simulink model "code_gen_HeadingHold"  (Simulink 7.5)
settings: Solver=FixedStepDiscrete  SolverMode=SingleTasking  StartTime=0.0  StopTime=10.0  FixedStep=0.01  RelTol=1e-3
InitFcn:
  | boat_constants
values from neighbouring files (symbols this model uses):
  figure8_waypoints = int32([ ... (first row only)    [boat_constants.m]
  OC2max = 49999    [boat_constants.m]    (also in simulation_constants.m)
  sampling_waypoints = int32([ ... (first row only)    [boat_constants.m]
  T_step = 0.01    [boat_constants.m]    (also in common.m)
  test_waypoints = int32([ ... (first row only)    [boat_constants.m]
undefined symbols (not defined in the file or in its folder): clearGpsData, clearSensorData, cpInitCommunications, DataEEInitAndClear, DataEEWrite, DiscIntNeverNeededParam, ecan1_buffered_transmit_matlab, ecan1_error_status_matlab, ecan1_init, ecan1_receive_matlab, getGpsData, getSensorData, Init_onlyOnce, Init_Reset, initCalibrationRange, initGps, processNewCommData, processNewGpsData, setHilMode, u1, u2, uart1EnqueueStateData, uart2EnqueueActuatorData, y1
libraries: simulink x85, dsPICdrivers x44, uSimLib x6, simulink_need_slupdate x4, aerolibconvert2 x2
(part 1 of 6)
CloseFcn:
  | rtwprivate ssgencode ModelCloseRequest code_gen
settings Model: Creator=bwmairs  LastModifiedBy=Bryant  BufferReuse=off
settings OptimizationCC: InlineParams=on  InlineInvariantSignals=on  OptimizeBlockIOStorage=off  BufferReuse=off  ExpressionFolding=off  LocalBlockOutputs=off  ZeroExternalMemoryAtStartup=off  ZeroInternalMemoryAtStartup=off  NoFixptDivByZeroProtection=on  EfficientFloat2IntCast=on  OptimizeModelRefInitCode=on
settings DebuggingCC: ReadBeforeWriteMsg=DisableAll  WriteAfterWriteMsg=DisableAll  WriteAfterReadMsg=DisableAll  ParameterOverflowMsg=warning  UniqueDataStoreMsg=error
settings HardwareCC: ProdBitPerInt=16  ProdIntDivRoundTo=Zero  ProdEndianess=LittleEndian  ProdWordSize=16  ProdHWDeviceType=16-bit Generic
settings RTWCC: SystemTargetFile=dspic.tlc  MakeCommand=make_CreateMPLAB  TemplateMakefile=dspic_pic30_gcc.tmf  PostCodeGenCommand=dsPIC_Compile()  Description=Embedded Target for Microchip dsPIC (real-time)  ProcessScript=dspic_make_rtw_hook  RTWCompilerOptimization=On
settings RTWCC: CustomSource=|
  | ../../../ECAN_dspic/circBuffer.c
  | ../../../ECAN_dspic/ecanFunctions.c
  | clib/gps.c
  | clib/commProtocol.c
  | clib/uart1.c
  | clib/uart2.c
  | clib/DEE.c
  | clib/DEES.s
  | clib/misc.c
settings CodeAppCC: IgnoreCustomStorageClasses=off  IgnoreTestpoints=on
settings STFCustomTargetCC: TargetFunctionLibrary=C89/C90 (ANSI)  IncludeMdlTerminateFcn=off  CombineOutputUpdateFcns=on  SuppressErrorStatus=on  ERTCustomFileBanners=on  SupportAbsoluteTime=off  SupportNonFinite=off  SupportComplex=off  SupportContinuousTime=off  SupportNonInlinedSFcns=off  SystemTargetFile=dspic.tlc
settings ERTTargetCC: TargetFunctionLibrary=C89/C90 (ANSI)  MultiwordLength=2048  ParMdlRefBuildCompliant=off  CompOptLevelCompliant=off  IncludeMdlTerminateFcn=off  SuppressErrorStatus=on  ERTFirstTimeCompliant=off  SupportAbsoluteTime=off  SupportNonFinite=off  SupportComplex=off  ModelStepFunctionPrototypeControlCompliant=off  CPPClassGenCompliant=off  ExtModeMexFile=ext_serial_win32_comm  InlinedParameterPlacement=NonHierarchical  ERTSrcFileBannerTemplate=dsPIC_code_template.cgt  ERTHdrFileBannerTemplate=dsPIC_code_template.cgt  ERTDataSrcFileTemplate=dsPIC_code_template.cgt  ERTDataHdrFileTemplate=dsPIC_code_template.cgt  ERTCustomFileTemplate=dsPIC_main.tlc
settings CustomProperty: DataType=string  Value=C:\PROGRA~1\MATLAB\R2010a\bin\win64\gmake

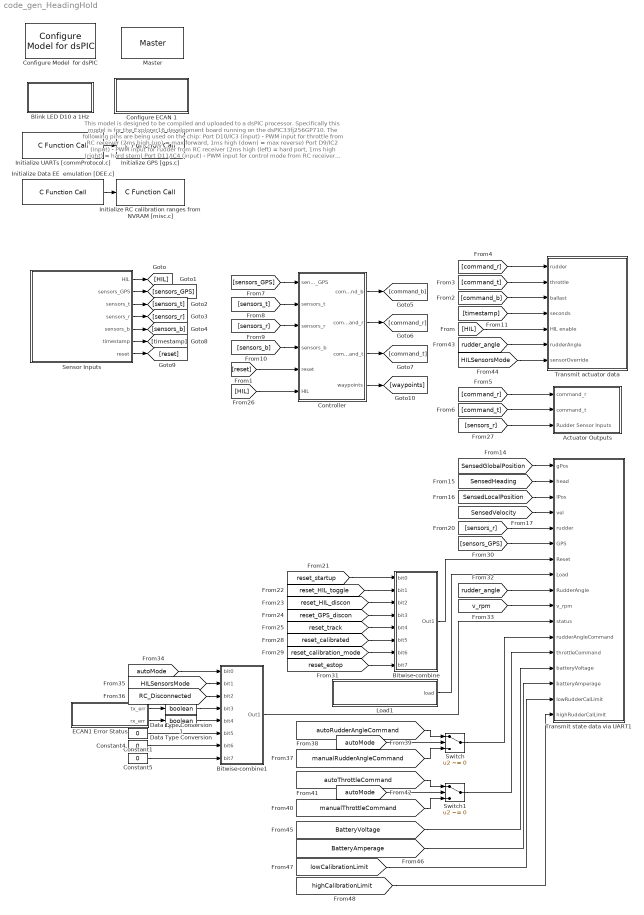
== system code_gen_HeadingHold ==
  note: This model is designed to be compiled and uploaded to a dsPIC processor.
      | Specifically this model is for the Explorer16 development board running on
      | the dsPIC33fj256GP710. The following pins are being used on the chip:
      | Port D10/IC3 (input) - PWM input for throttle from RC receiver (2ms high (up) = max forward, 1ms high (down) = max reverse)
      | Port D9/IC2 (input) - PWM input for rudder from RC receiver (2ms high (left) = hard port, 1ms high (right) = hard stern)
      | Port D11/IC4 (input) - PWM input for control mode from RC receiver (2ms high (down) = manual control, 1ms high (up) = auto. control)
      | Port D15/IC8 (input) - PWM input for track control from RC receiver (2ms high (left) = resetTrack, 1ms high (right) = nextTrack)
      | Port C2 (input) - Port hall effect sensor
      | Port G3 (input) - Starboard hall effect sensor
      | Port B4/AN4 (input) - ADC input for the TC1047 temperature sensor
      | Port B0/AN0 (input) - Potentiometer measuring position for the rudder
      | Port OC2/RD1 (output) - Step output for the rudder driver board
      | Port G9 (output) - Enable output for the rudder driver board, wired low
      | Port D5 (output) - Direction output for the rudder driver board (low = rudder turns to port)
      | Ports F0/1 (in/out) - Pins required for the ECAN1 peripheral. This is used for controlling the propeller motor.
      | Ports F4/5 (in/out) - Pins required for the UART2 peripheral. This is used for HIL data or GPS input.
      | Port A7 (out) - 1Hz pulses to blink a status LED
      | Port A0 (out) - High when in reset (drives an LED on the explorer16)
      | Port A1 (out) - High when in HIL mode (drives an LED on the explorer16)
      | Port A2 (out) - High when autonomous mode is enabled. (drives an LED on the explorer16)
      | Port F2/3 (in/out) - UART1 transmission line.
      | Port B9/11 (in/in) - ADC inputs for voltage (B9) and current (B11) sensor
      |
      | A failsafe has been implemented to detect the loss of an RC connection. It reduces propeller speed to zero and
      | disables rudder control.
      |
      | Switching between the autonomous controller and manual control involves using the landing gear channel. When
      | it's enabled, it's under autonomous control. This can only be changed when the RC transmitter is on and connected and
      | is never changed otherwise.
  Actuator Outputs : Subsystem
  Bitwise-combine : Subsystem
  Bitwise-combine1 : Subsystem
  Blink LED D10 a 1Hz : Subsystem
      mask Display: disp('blink');
  Configure ECAN 1 : Subsystem  mask(Initialize ECAN 1){frame_setting=off, mode=Normal, dma_rx_chan=2, dma_tx_chan=0, baud=250000, ps1=8, pd=5, ps2=6, sjw=4, tq=20, triple_sample=on, dma_buf_size=8 buffers, rx_bufs=[1], tx_bufs=[0], buf_0_tx_pri=Highest, buf_0_rte=No, buf_1_tx_pri=Highest, buf_1_rte=No, buf_2_tx_pri=Lowest, buf_2_rte=No, buf_3_tx_pri=Lowest, buf_3_rte=No, buf_4_tx_pri=Lowest, buf_4_rte=No, buf_5_tx_pri=Lowest, buf_5_rte=No, buf_6_tx_pri=Lowest, buf_6_rte=No, buf_7_tx_pri=Lowest, buf_7_rte=No, mask_0=0, mask_0_mide=Match std or ext, mask_1=0, mask_1_mide=Match std or ext, mask_2=0, mask_2_mide=Match std or ext, filters=[0], filter_0=0, filter_0_mask=0, filter_0_exide=Match only standard, filter_0_buf=1, filter_1=hex2dec('401'), filter_1_mask=0, filter_1_exide=Match only standard, filter_1_buf=2, filter_2=hex2dec('402'), filter_2_mask=0, filter_2_exide=Match only standard, filter_2_buf=3, filter_3=0, filter_3_mask=0, filter_3_exide=Match only standard, filter_3_buf=0, filter_4=0, filter_4_mask=0, filter_4_exide=Match only standard, filter_4_buf=0, filter_5=0, filter_5_mask=0, filter_5_exide=Match only standard, filter_5_buf=0, filter_6=0, filter_6_mask=0, filter_6_exide=Match only standard, filter_6_buf=0, filter_7=0, filter_7_mask=0, filter_7_exide=Match only standard, filter_7_buf=0, filter_8=0, filter_8_mask=0, filter_8_exide=Match only standard, filter_8_buf=0, filter_9=0, filter_9_mask=<empty>, filter_9_exide=Match only standard, filter_9_buf=0, filter_10=0, filter_10_mask=0, filter_10_exide=Match only standard, filter_10_buf=0, filter_11=0, filter_11_mask=0, filter_11_exide=Match only standard, filter_11_buf=0, filter_12=0, filter_12_mask=0, filter_12_exide=Match only standard, filter_12_buf=0, filter_13=0, filter_13_mask=0, filter_13_exide=Match only standard, filter_13_buf=0, filter_14=0, filter_14_mask=0, filter_14_exide=Match only standard, filter_14_buf=0, filter_15=0, filter_15_mask=0, filter_15_exide=Match only standard, filter_15_buf=0}
      mask prompts: frame_setting "Extended Frames (Standard if unchecked)"; dma_rx_chan "DMA Reception Channel"; dma_tx_chan "DMA Transmission Channel"; baud "Baud Rate (bps)"; ps1 "Phase Segment 1"; pd "Propagation Delay"; ps2 "Phase Segment 2"; sjw "Sync Jump Width"; tq "Time Quanta"; triple_sample "Triple-sample"; dma_buf_size "DMA Buffer Size"; rx_bufs "Reception Buffers"; tx_bufs "Transmission Buffers"; buf_0_tx_pri "Buffer 0 Transmission Priority"; buf_0_rte "Buffer 0 Remote Transmit Enable"; buf_1_tx_pri "Buffer 1 Transmission Priority"; buf_1_rte "Buffer 1 Remote Transmit Enable"; buf_2_tx_pri "Buffer 2 Transmission Priority"; buf_2_rte "Buffer 2 Remote Transmit Enable"; buf_3_tx_pri "Buffer 3 Transmission Priority"; buf_3_rte "Buffer 3 Remote Transmit Enable"; buf_4_tx_pri "Buffer 4 Transmission Priority"; buf_4_rte "Buffer 4 Remote Transmit Enable"; buf_5_tx_pri "Buffer 5 Transmission Priority"; buf_5_rte "Buffer 5 Remote Transmit Enable"; buf_6_tx_pri "Buffer 6 Transmission Priority"; buf_6_rte "Buffer 6 Remote Transmit Enable"; buf_7_tx_pri "Buffer 7 Transmission Priority"; buf_7_rte "Buffer 7 Remote Transmit Enable"; mask_0 "Mask 0"; mask_0_mide "Mask 0 Receive Mode"; mask_1 "Mask 1"; mask_1_mide "Mask 1 Receive Mode"; mask_2 "Mask 2"; mask_2_mide "Mask 2 Receive Mode"; filter_0 "Filter 0"; filter_0_mask "Filter 0 Mask"; filter_0_exide "Filter 0 Mode"; filter_0_buf "Filter 0 Buffer"; filter_1 "Filter 1"; filter_1_mask "Filter 1 Mask"; filter_1_exide "Filter 1 Mode"; filter_1_buf "Filter 1 Buffer"; filter_2 "Filter 2"; filter_2_mask "Filter 2 Mask"; filter_2_exide "Filter 2 Mode"; filter_2_buf "Filter 2 Buffer"; filter_3 "Filter 3"; filter_3_mask "Filter 3 Mask"; filter_3_exide "Filter 3 Mode"; filter_3_buf "Filter 3 Buffer"; filter_4 "Filter 4"; filter_4_mask "Filter 4 Mask"; filter_4_exide "Filter 4 Mode"; filter_4_buf "Filter 4 Buffer"; filter_5 "Filter 5"; filter_5_mask "Filter 5 Mask"; filter_5_exide "Filter 5 Mode"; filter_5_buf "Filter 5 Buffer"; filter_6 "Filter 6"; filter_6_mask "Filter 6 Mask"; filter_6_exide "Filter 6 Mode"; filter_6_buf "Filter 6 Buffer"; filter_7 "Filter 7"; filter_7_mask "Filter 7 Mask"; filter_7_exide "Filter 7 Mode"; filter_7_buf "Filter 7 Buffer"; filter_8 "Filter 8"; filter_8_mask "Filter 8 Mask"; filter_8_exide "Filter 8 Mode"; filter_8_buf "Filter 8 Buffer"; filter_9 "Filter 9"; filter_9_mask "Filter 9 Mask"; filter_9_exide "Filter 9 Mode"; filter_9_buf "Filter 9 Buffer"; filter_10 "Filter 10"; filter_10_mask "Filter 10 Mask"; filter_10_exide "Filter 10 Mode"; filter_10_buf "Filter 10 Buffer"; filter_11 "Filter 11"; filter_11_mask "Filter 11 Mask"; filter_11_exide "Filter 11 Mode"; filter_11_buf "Filter 11 Buffer"; filter_12 "Filter 12"; filter_12_mask "Filter 12 Mask"; filter_12_exide "Filter 12 Mode"; filter_12_buf "Filter 12 Buffer"; filter_13 "Filter 13"; filter_13_mask "Filter 13 Mask"; filter_13_exide "Filter 13 Mode"; filter_13_buf "Filter 13 Buffer"; filter_14 "Filter 14"; filter_14_mask "Filter 14 Mask"; filter_14_exide "Filter 14 Mode"; filter_14_buf "Filter 14 Buffer"; filter_15 "Filter 15"; filter_15_mask "Filter 15 Mask"; filter_15_exide "Filter 15 Mode"; filter_15_buf "Filter 15 Buffer"
      mask help: Initializes the ECAN 1 module on the dsPIC33f. Allows for configuration of almost all ECAN options to produce a usable system.
      mask init:
      | parameters = uint16(zeros(53,1));
      | 
      | %% Generate parameter 1
      | parameters(1) = frame_setting;
      | mode_id = 0;
      | switch mode
      |     case 'Disabled'
      |         mode_id = 1;
      |     case 'Loopback'
      |         mode_id = 2;
      |     case 'Listen only'
      |         mode_id = 3;
      |     case 'Listen all'
      |         mode_id = 7;
      | end
      | parameters(1) = bitor(parameters(1), bitshift(mode_id, 2));
      | parameters(1) = bitor(parameters(1), bitshift(dma_rx_chan, 5));
      | parameters(1) = bitor(parameters(1), bitshift(dma_tx_chan, 8));
      | 
      | %% Generate parameter 2
      | parameters(2) = baud / 100;
      | 
      | %% Generate parameter 3
      | h = find_system(bdroot(gcb),'FollowLinks','on','LookUnderMasks','all','Tag','dsPIC_MASTER');
      | fcy = 0;
      | if ~isempty(h)
      |     %OverrideFcy = strcmp(get_param(h{1},'OverrideFcy'),'on');
      |     %if (OverrideFcy == 1)
      |     %    fcy = str2num(get_param(h{1},'NewFcy'));     %% overridded fcy
      |     %else
      |         fcy = str2num(get_param(h{1},'fcy'));
      |     %end 
      | end
      | parameters(3) = fcy / 1000;
      | 
      | %% Generate parameter 4
      | parameters(4) = ps1 - 1;
      | parameters(4) = bitor(parameters(4), bitshift(pd - 1, 3));
      | parameters(4) = bitor(parameters(4), bitshift(ps2 - 1, 6));
      | parameters(4) = bitor(parameters(4), bitshift(sjw - 1, 9));
      | if triple_sample == 1
      |     parameters(4) = bitset(parameters(4),12);
      | end
      | 
      | %% Generate parameter 5
      | for k = 1:length(filters)
      |     parameters(5) = bitset(parameters(5),filters(k)+1);
      | end;
      | 
      | % Map filter mask values into proper values
      | filter_masks = [filter_0_mask; filter_1_mask; filter_2_mask; filter_3_mask; filter_4_mask; filter_5_mask; filter_6_mask; filter_7_mask; filter_8_mask; filter_9_mask; filter_10_mask; filter_11_mask; filter_12_mask; filter_13_mask; filter_14_mask; filter_15_mask;];
      | filter_masks = filter_masks - 2;
      | filter_masks(filter_masks == -1) = 3;
      | 
      | %% Generate parameters 6 and 7
      | for k = 1:length(filters);
      |     filter = filters(k) + 1;
      |     if filter < 9
      |         parameters(6) = bitor(parameters(6), bitshift(filter_masks(filter),2*(filter-1)));
      |     else
      |         parameters(7) = bitor(parameters(7), bitshift(filter_masks(filter),2*(filter-9)));
      |     end
      | end
      | 
      | % Generate parameters 8 and 9
      | parameters(8) = bitshift(bitand(mask_0,hex2dec('18000000')),-27); % EID17-16
      | parameters(8) = bitor(parameters(8), bitshift(bitand(mask_0,hex2dec('7FF')), 5)); % SID
      | parameters(8) = bitor(parameters(8), bitshift(mask_0_mide - 1, 3)); % MIDE
      | parameters(9) = bitshift(bitand(mask_0,hex2dec('7FFF800')),-11); % EID15-0
      | 
      | %% Generate parameters 10 and 11
      | parameters(10) = bitshift(bitand(mask_1,hex2dec('18000000')),-27); % EID17-16
      | parameters(10) = bitor(parameters(10), bitshift(bitand(mask_1,hex2dec('7FF')), 5)); % SID
      | parameters(10) = bitor(parameters(10), bitshift(mask_1_mide - 1, 3)); % MIDE
      | parameters(11) = bitshift(bitand(mask_1,hex2dec('7FFF800')),-11); % EID15-0
      | 
      | %% Generate parameters 12 and 13
      | parameters(12) = bitshift(bitand(mask_2,hex2dec('18000000')),-27); % EID17-16
      | parameters(12) = bitor(parameters(12), bitshift(bitand(mask_2,hex2dec('7FF')), 5)); % SID
      | parameters(12) = bitor(parameters(12), bitshift(mask_2_mide - 1, 3)); % MIDE
      | parameters(13) = bitshift(bitand(mask_2,hex2dec('7FFF800')),-11); % EID15-0
      | 
      | % Generate parameters 14-17
      | buf_priorities = [buf_0_tx_pri;buf_1_tx_pri;buf_2_tx_pri;buf_3_tx_pri;buf_4_tx_pri;buf_5_tx_pri;buf_6_tx_pri;buf_7_tx_pri] - 1;
      | buf_rtes = [buf_0_rte;buf_1_rte;buf_2_rte;buf_3_rte;buf_4_rte;buf_5_rte;buf_6_rte;buf_7_rte] - 1;
      | 
      | % Create a vector of chars to modify
      | regs = uint16(zeros(8,1));
      | 
      | % Go through all enabled transmission buffers setting appropriate bits
      | for b = 1:size(tx_bufs,1)
      |     
      |     index = tx_bufs(b) + 1;
      |     
      |     % Set transmission bit
      |     regs(index) = bitset(regs(index),8);
      | 
      |     % Set priority bits
      |     regs(index) = bitor(regs(index), buf_priorities(index));
      | 
      |     % Set remote transmit enable bits
      |     if buf_rtes(index) == 1
      |         regs(index) = bitset(regs(index),3);
      |     end
      | end
      | 
      | for b = 1:size(rx_bufs,1)
      |     
      |     index = rx_bufs(b) + 1;
      | 
      |     % Set priority bits
      |     regs(index) = bitor(regs(index), buf_priorities(index));
      | 
      |     % Set remote transmit enable bits
      |     if buf_rtes(index) == 1
      |         regs(index) = bitset(regs(index),3);
      |     end
      | end
      | 
      | % Map our matrix into registers
      | parameters(14) = bitor(bitshift(regs(2),8), regs(1));
      | parameters(15) = bitor(bitshift(regs(4),8), regs(3));
      | parameters(16) = bitor(bitshift(regs(6),8), regs(5));
      | parameters(17) = bitor(bitshift(regs(8),8), regs(7));
      | 
      | % Map the filter buffer values to corresponding bit values
      | filter_buffers = [filter_0_buf; filter_1_buf; filter_2_buf; filter_3_buf; filter_4_buf; filter_5_buf; filter_6_buf; filter_7_buf; filter_8_buf; filter_9_buf; filter_10_buf; filter_11_buf; filter_12_buf; filter_13_buf; filter_14_buf; filter_15_buf;];
      | filter_buffers = filter_buffers - 1;
      | 
      | %% Generate parameter 18
      | if bitget(parameters(5),1) == 1
      |     parameters(18) = filter_buffers(1);
      | end
      | if bitget(parameters(5),2) == 1
      |     parameters(18) = bitor(parameters(18), bitshift(filter_buffers(2), 4));
      | end
      | if bitget(parameters(5),3) == 1
      |     parameters(18) = bitor(parameters(18), bitshift(filter_buffers(3), 8));
      | end
      | if bitget(parameters(5),4) == 1
      |     parameters(18) = bitor(parameters(18), bitshift(filter_buffers(4), 12));
      | end
      | 
      | %% Generate parameter 19
      | if bitget(parameters(5),5) == 1
      |     parameters(19) = filter_buffers(5);
      | end
      | if bitget(parameters(5),6) == 1
      |     parameters(19) = bitor(parameters(19), bitshift(filter_buffers(6), 4));
      | end
      | if bitget(parameters(5),7) == 1
      |     parameters(19) = bitor(parameters(19), bitshift(filter_buffers(7), 8));
      | end
      | if bitget(parameters(5),8) == 1
      |     parameters(19) = bitor(parameters(19), bitshift(filter_buffers(8), 12));
      | end
      | 
      | %% Generate parameter 20
      | if bitget(parameters(5),9) == 1
      |     parameters(20) = filter_buffers(9);
      | end
      | if bitget(parameters(5),10) == 1
      |     parameters(20) = bitor(parameters(20), bitshift(filter_buffers(10), 4));
      | end
      | if bitget(parameters(5),11) == 1
      |     parameters(20) = bitor(parameters(20), bitshift(filter_buffers(11), 8));
      | end
      | if bitget(parameters(5),12) == 1
      |     parameters(20) = bitor(parameters(20), bitshift(filter_buffers(12), 12));
      | end
      | 
      | %% Generate parameter 21
      | if bitget(parameters(5),13) == 1
      |     parameters(21) = filter_buffers(13);
      | end
      | if bitget(parameters(5),14) == 1
      |     parameters(21) = bitor(parameters(21), bitshift(filter_buffers(14), 4));
      | end
      | if bitget(parameters(5),15) == 1
      |     parameters(21) = bitor(parameters(21), bitshift(filter_buffers(15), 8));
      | end
      | if bitget(parameters(5),16) == 1
      |     parameters(21) = bitor(parameters(21), bitshift(filter_buffers(16), 12));
      | end
      | 
      | % Generate parameters 22 and 23
      | parameters(22) = bitshift(bitand(filter_0,hex2dec('18000000')),-27); % EID17-16
      | parameters(22) = bitor(parameters(22), bitshift(bitand(filter_0,hex2dec('7FF')), 5)); % SID
      | parameters(22) = bitor(parameters(22), bitshift(filter_0_exide - 1, 3)); % EXIDE
      | parameters(23) = bitshift(bitand(uint32(filter_0),hex2dec('7FFF800')),-11); % EID15-0
      | 
      | %% Generate parameters 24 and 25
      | parameters(24) = bitshift(bitand(filter_1,hex2dec('18000000')),-27); % EID17-16
      | parameters(24) = bitor(parameters(24), bitshift(bitand(filter_1,hex2dec('7FF')), 5)); % SID
      | parameters(24) = bitor(parameters(24), bitshift(filter_1_exide - 1, 3)); % EXIDE
      | parameters(25) = bitshift(bitand(uint32(filter_1),hex2dec('7FFF800')),-11); % EID15-0
      | 
      | %% Generate parameters 26 and 27
      | parameters(26) = bitshift(bitand(filter_2,hex2dec('18000000')),-27); % EID17-16
      | parameters(26) = bitor(parameters(26), bitshift(bitand(filter_2,hex2dec('7FF')), 5)); % SID
      | parameters(26) = bitor(parameters(26), bitshift(filter_2_exide - 1, 3)); % EXIDE
      | parameters(27) = bitshift(bitand(uint32(filter_2),hex2dec('7FFF800')),-11); % EID15-0
      | 
      | %% Generate parameters 28 and 29
      | parameters(28) = bitshift(bitand(filter_3,hex2dec('18000000')),-27); % EID17-16
      | parameters(28) = bitor(parameters(28), bitshift(bitand(filter_3,hex2dec('7FF')), 5)); % SID
      | parameters(28) = bitor(parameters(28), bitshift(filter_3_exide - 1, 3)); % EXIDE
      | parameters(29) = bitshift(bitand(uint32(filter_3),hex2dec('7FFF800')),-11); % EID15-0
      | 
      | %% Generate parameters 30 and 31
      | parameters(30) = bitshift(bitand(filter_4,hex2dec('18000000')),-27); % EID17-16
      | parameters(30) = bitor(parameters(30), bitshift(bitand(filter_4,hex2dec('7FF')), 5)); % SID
      | parameters(30) = bitor(parameters(30), bitshift(filter_4_exide - 1, 3)); % EXIDE
      | parameters(31) = bitshift(bitand(uint32(filter_4),hex2dec('7FFF800')),-11); % EID15-0
      | 
      | %% Generate parameters 32 and 33
      | parameters(32) = bitshift(bitand(filter_5,hex2dec('18000000')),-27); % EID17-16
      | parameters(32) = bitor(parameters(32), bitshift(bitand(filter_5,hex2dec('7FF')), 5)); % SID
      | parameters(32) = bitor(parameters(32), bitshift(filter_5_exide - 1, 3)); % EXIDE
      | parameters(33) = bitshift(bitand(uint32(filter_5),hex2dec('7FFF800')),-11); % EID15-0
      | 
      | %% Generate parameters 34 and 35
      | parameters(34) = bitshift(bitand(filter_6,hex2dec('18000000')),-27); % EID17-16
      | parameters(34) = bitor(parameters(34), bitshift(bitand(filter_6,hex2dec('7FF')), 5)); % SID
      | parameters(34) = bitor(parameters(34), bitshift(filter_6_exide - 1, 3)); % EXIDE
      | parameters(35) = bitshift(bitand(uint32(filter_6),hex2dec('7FFF800')),-11); % EID15-0
      | 
      | %% Generate parameters 36 and 37
      | parameters(36) = bitshift(bitand(filter_7,hex2dec('18000000')),-27); % EID17-16
      | parameters(36) = bitor(parameters(36), bitshift(bitand(filter_7,hex2dec('7FF')), 5)); % SID
      | parameters(36) = bitor(parameters(36), bitshift(filter_7_exide - 1, 3)); % EXIDE
      | parameters(37) = bitshift(bitand(uint32(filter_7),hex2dec('7FFF800')),-11); % EID15-0
      | 
      | %% Generate parameters 38 and 39
      | parameters(38) = bitshift(bitand(filter_8,hex2dec('18000000')),-27); % EID17-16
      | parameters(38) = bitor(parameters(38), bitshift(bitand(filter_8,hex2dec('7FF')), 5)); % SID
      | parameters(38) = bitor(parameters(38), bitshift(filter_8_exide - 1, 3)); % EXIDE
      | parameters(39) = bitshift(bitand(uint32(filter_8),hex2dec('7FFF800')),-11); % EID15-0
      | 
      | %% Generate parameters 40 and 41
      | parameters(40) = bitshift(bitand(filter_9,hex2dec('18000000')),-27); % EID17-16
      | parameters(40) = bitor(parameters(40), bitshift(bitand(filter_9,hex2dec('7FF')), 5)); % SID
      | parameters(40) = bitor(parameters(40), bitshift(filter_9_exide - 1, 3)); % EXIDE
      | parameters(41) = bitshift(bitand(uint32(filter_9),hex2dec('7FFF800')),-11); % EID15-0
      | 
      | %% Generate parameters 42 and 43
      | parameters(42) = bitshift(bitand(filter_10,hex2dec('18000000')),-27); % EID17-16
      | parameters(42) = bitor(parameters(42), bitshift(bitand(filter_10,hex2dec('7FF')), 5)); % SID
      | parameters(42) = bitor(parameters(42), bitshift(filter_10_exide - 1, 3)); % EXIDE
      | parameters(43) = bitshift(bitand(uint32(filter_10),hex2dec('7FFF800')),-11); % EID15-0
      | 
      | %% Generate parameters 44 and 45
      | parameters(44) = bitshift(bitand(filter_11,hex2dec('18000000')),-27); % EID17-16
      | parameters(44) = bitor(parameters(44), bitshift(bitand(filter_11,hex2dec('7FF')), 5)); % SID
      | parameters(44) = bitor(parameters(44), bitshift(filter_11_exide - 1, 3)); % EXIDE
      | parameters(45) = bitshift(bitand(uint32(filter_11),hex2dec('7FFF800')),-11); % EID15-0
      | 
      | %% Generate parameters 46 and 47
      | parameters(46) = bitshift(bitand(filter_12,hex2dec('18000000')),-27); % EID17-16
      | parameters(46) = bitor(parameters(46), bitshift(bitand(filter_12,hex2dec('7FF')), 5)); % SID
      | parameters(46) = bitor(parameters(46), bitshift(filter_12_exide - 1, 3)); % EXIDE
      | parameters(47) = bitshift(bitand(uint32(filter_12),hex2dec('7FFF800')),-11); % EID15-0
      | 
      | %% Generate parameters 48 and 49
      | parameters(48) = bitshift(bitand(filter_13,hex2dec('18000000')),-27); % EID17-16
      | parameters(48) = bitor(parameters(48), bitshift(bitand(filter_13,hex2dec('7FF')), 5)); % SID
      | parameters(48) = bitor(parameters(48), bitshift(filter_13_exide - 1, 3)); % EXIDE
      | parameters(49) = bitshift(bitand(uint32(filter_13),hex2dec('7FFF800')),-11); % EID15-0
      | 
      | %% Generate parameters 50 and 51
      | parameters(50) = bitshift(bitand(filter_14,hex2dec('18000000')),-27); % EID17-16
      | parameters(50) = bitor(parameters(50), bitshift(bitand(filter_14,hex2dec('7FF')), 5)); % SID
      | parameters(50) = bitor(parameters(50), bitshift(filter_14_exide - 1, 3)); % EXIDE
      | parameters(51) = bitshift(bitand(uint32(filter_14),hex2dec('7FFF800')),-11); % EID15-0
      | 
      | %% Generate parameters 52 and 53
      | parameters(52) = bitshift(bitand(filter_15,hex2dec('18000000')),-27); % EID17-16
      | parameters(52) = bitor(parameters(52), bitshift(bitand(filter_15,hex2dec('7FF')), 5)); % SID
      | parameters(52) = bitor(parameters(52), bitshift(filter_15_exide - 1, 3)); % EXIDE
      | parameters(53) = bitshift(bitand(uint32(filter_15),hex2dec('7FFF800')),-11); % EID15-0
      mask StyleString: checkbox,popup(Disabled|Listen all|Listen only|Loopback|Normal),edit,edit,edit,edit,edit,edit,popup(1|2|3|4),edit,checkbox,popup(4 buffers|6 buffers|8 buffers|12 buffers|16 buffers|24 buffers|32 buffers),edit,edit,popup(Lowest|Low|High|Highest),popup(No|Yes),popup(Lowest|Low|High|Highest),popup(No|Yes),popup(Lowest|Low|High|Highest),popup(No|Yes),popup(Lowest|Low|High|Highest),popup(No|Yes),popup(Lowest|Low|High|Highest),popup(No|Yes),popup(Lowest|Low|High|Highest),popup(No|Yes),popup(Lowest|Low|High|Highest),popup(No|Yes),popup(Lowest|Low|High|Highest),popup(No|Yes),edit,popup(Match std or ext|Obey filter mode),edit,popup(Match std or ext|Obey filter mode),edit,popup(Match std or ext|Obey filter mode),edit,edit,popup(--|0|1|2),popup(Match only standard|Match only extended),popup(0|1|2|3|4|5|6|7|8|9|10|11|12|13|14|FIFO),edit,popup(--|0|1|2),popup(Match only standard|Match only extended),popup(0|1|2|3|4|5|6|7|8|9|10|11|12|13|14|FIFO),edit,popup(--|0|1|2),popup(Match only standard|Match only extended),popup(0|1|2|3|4|5|6|7|8|9|10|11|12|13|14|FIFO),edit,popup(--|0|1|2),popup(Match only standard|Match only extended),popup(0|1|2|3|4|5|6|7|8|9|10|11|12|13|14|FIFO),edit,popup(--|0|1|2),popup(Match only standard|Match only extended),popup(0|1|2|3|4|5|6|7|8|9|10|11|12|13|14|FIFO),edit,popup(--|0|1|2),popup(Match only standard|Match only extended),popup(0|1|2|3|4|5|6|7|8|9|10|11|12|13|14|FIFO),edit,popup(--|0|1|2),popup(Match only standard|Match only extended),popup(0|1|2|3|4|5|6|7|8|9|10|11|12|13|14|FIFO),edit,popup(--|0|1|2),popup(Match only standard|Match only extended),popup(0|1|2|3|4|5|6|7|8|9|10|11|12|13|14|FIFO),edit,popup(--|0|1|2),popup(Match only standard|Match only extended),popup(0|1|2|3|4|5|6|7|8|9|10|11|12|13|14|FIFO),edit,popup(<empty>),popup(Match only standard|Match only extended),popup(0|1|2|3|4|5|6|7|8|9|10|11|12|13|14|FIFO),edit,popup(--|0|1|2),popup(Match only standard|Match only extended),popup(0|1|2|3|4|5|6|7|8|9|10|11|12|13|14|FIFO),edit,popup(--|0|1|2),popup(Match only standard|Match only extended),popup(0|1|2|3|4|5|6|7|8|9|10|11|12|13|14|FIFO),edit,popup(--|0|1|2),popup(Match only standard|Match only extended),popup(0|1|2|3|4|5|6|7|8|9|10|11|12|13|14|FIFO),edit,popup(--|0|1|2),popup(Match only standard|Match only extended),popup(0|1|2|3|4|5|6|7|8|9|10|11|12|13|14|FIFO),edit,popup(--|0|1|2),popup(Match only standard|Match only extended),popup(0|1|2|3|4|5|6|7|8|9|10|11|12|13|14|FIFO),edit,popup(--|0|1|2),popup(Match only standard|Match only extended),popup(0|1|2|3|4|5|6|7|8|9|10|11|12|13|14|FIFO)
      mask CallbackString:
      | |||||tq = 1 + str2num(get_param(gcb, 'ps1')) + str2num(get_param(gcb, 'pd')) + str2num(get_param(gcb, 'ps2'));
      | set_param(gcb, 'tq', int2str(tq));|tq = 1 + str2num(get_param(gcb, 'ps1')) + str2num(get_param(gcb, 'pd')) + str2num(get_param(gcb, 'ps2'));
      | set_param(gcb, 'tq', int2str(tq));|tq = 1 + str2num(get_param(gcb, 'ps1')) + str2num(get_param(gcb, 'pd')) + str2num(get_param(gcb, 'ps2'));
      | set_param(gcb, 'tq', int2str(tq));||||||filters = eval(get_param(gcb,'tx_bufs'));
      | mVisibilities = get_param(gcb,'MaskVisibilities');
      | mNames = get_param(gcb,'MaskNames');
      | for i = 1:size(mNames);
      | 	n = mNames{i};
      |     if size(n,2) > 4 && strcmp(n(1:4), 'buf_') == 1
      |         filterNumber = sscanf(n, 'buf_%d');
      |         if isempty(find(filters == filterNumber, 1)) == 0
      |              mVisibilities{i} = 'on';
      |         else
      |              mVisibilities{i} = 'off';
      |         end
      |     end
      | end
      | set_param(gcb, 'MaskVisibilities', mVisibilities);|||||||||||||||||||||||filters = eval(get_param(gcb,'filters'));
      | mVisibilities = get_param(gcb,'MaskVisibilities');
      | mNames = get_param(gcb,'MaskNames');
      | for i = 1:size(mNames);
      | 	n = mNames{i};
      |     if size(n,2) > 7 && strcmp(n(1:7), 'filter_') == 1
      |         filterNumber = sscanf(n, 'filter_%d');
      |         if isempty(find(filters == filterNumber, 1)) == 0
      |              mVisibilities{i} = 'on';
      |         else
      |              mVisibilities{i} = 'off';
      |         end
      |     end
      | end
      | set_param(gcb, 'MaskVisibilities', mVisibilities);||||||||||||||||||||||||||||||||||||||||||||||||||||||||||||||||
      mask Display: text(0.5,0.5,'Configure ECAN1','horizontalAlignment','center','verticalAlignment','middle');
  Configure Model  for dsPIC : dsPICdrivers/Simulink Configuration/Configure Model  for dsPIC
  Constant1 : Constant  Value=0  OutDataTypeMode=uint8  OutDataType=fixdt(1, 16)  OutScaling=2^0  OutDataTypeStr=uint8
  Constant4 : Constant  Value=0  OutDataTypeMode=uint8  OutDataType=fixdt(1, 16)  OutScaling=2^0  OutDataTypeStr=uint8
  Constant5 : Constant  Value=0  OutDataTypeMode=uint8  OutDataType=fixdt(1, 16)  OutScaling=2^0  OutDataTypeStr=uint8
  Controller : Subsystem
  Data Type Conversion : DataTypeConversion  OutDataTypeMode=boolean  OutDataType=fixdt(1, 16)  OutScaling=2^0  OutDataTypeStr=boolean
  Data Type Conversion1 : DataTypeConversion  OutDataTypeMode=boolean  OutDataType=fixdt(1, 16)  OutScaling=2^0  OutDataTypeStr=boolean
  ECAN1 Error Status : Subsystem  mask(ECAN 1 Reception Block){ecan1_error_sample_time=.01}
      mask prompts: ecan1_error_sample_time "Sampling time"
      mask help:
      | This block will receive CAN messages over the ECAN1 peripheral on the dsPIC33f.
      | Outputs:
      | identifier - uint32 containing SID and EID
      | data - Variable-sized array (between 0 and 8) of uint8s
      | remote - boolean value specifying if this is a remote transmit request
      mask Display: disp('ECAN1 ERR');
  Initialize Data EE  emulation [DEE.c] : dsPICdrivers/OTHERS/C Function Call  Tag=dsPIC_dsPIC_CFunctionCall  FctUpdate=None  fctName='DataEEInitAndClear'  INPUT_SIZE=1  INPUT1=--  INPUT2=--  INPUT3=--  OUTPUT_SIZE=1  OUTPUT1=--  SampleTime=Inf  InputType=[]  OutputType=[]  FctDeclaration=extern void DataEEInitAndClear();  FctCall=DataEEInitAndClear();  OrderingInOutPopup=Output  FctStart=Start Function (Call once and only once)  FctStart_Name=DataEEInitAndClear  FctStart_Declaration=inline extern void DataEEInitAndClear();  FctStart_Call=DataEEInitAndClear();  FctInit=None  FctInit_Name=Init_Reset  FctInit_Declaration=inline extern void Init_Reset();  FctInit_Call=Init_Reset();  PinDigitalInput=[]  PinDigitalOutput=[]  AnalogueInput=[]
  Initialize GPS [gps.c] : dsPICdrivers/OTHERS/C Function Call  Tag=dsPIC_dsPIC_CFunctionCall  FctUpdate=None  fctName='initGps'  INPUT_SIZE=1  INPUT1=--  INPUT2=--  INPUT3=--  OUTPUT_SIZE=1  OUTPUT1=--  SampleTime=Inf  InputType=[]  OutputType=[]  FctDeclaration=extern void initGps();  FctCall=initGps();  OrderingInOutPopup=Input  FctStart=Start Function (Call once and only once)  FctStart_Name=initGps  FctStart_Declaration=inline extern void initGps();  FctStart_Call=initGps();  FctInit=None  FctInit_Name=Init_Reset  FctInit_Declaration=inline extern void Init_Reset();  FctInit_Call=Init_Reset();  PinDigitalInput=[]  PinDigitalOutput=[]  AnalogueInput=[]
  Initialize RC calibration ranges from NVRAM [misc.c] : dsPICdrivers/OTHERS/C Function Call  Tag=dsPIC_dsPIC_CFunctionCall  FctUpdate=None  fctName='initCalibrationRange'  INPUT_SIZE=1  INPUT1=--  INPUT2=--  INPUT3=--  OUTPUT_SIZE=1  OUTPUT1=--  SampleTime=Inf  InputType=[]  OutputType=[]  FctDeclaration=extern void initCalibrationRange();  FctCall=initCalibrationRange();  OrderingInOutPopup=Input  FctStart=Start Function (Call once and only once)  FctStart_Name=initCalibrationRange  FctStart_Declaration=inline extern void initCalibrationRange();  FctStart_Call=initCalibrationRange();  FctInit=None  FctInit_Name=Init_Reset  FctInit_Declaration=inline extern void Init_Reset();  FctInit_Call=Init_Reset();  PinDigitalInput=[]  PinDigitalOutput=[]  AnalogueInput=[]
  Initialize UARTs [commProtocol.c] : dsPICdrivers/OTHERS/C Function Call  Tag=dsPIC_dsPIC_CFunctionCall  FctUpdate=None  fctName=cpInitCommunications  INPUT_SIZE=1  INPUT1=--  INPUT2=--  INPUT3=--  OUTPUT_SIZE=1  OUTPUT1=--  SampleTime=Inf  InputType=[]  OutputType=[]  FctDeclaration=extern void cpInitCommunications();  FctCall=cpInitCommunications();  OrderingInOutPopup=Output  FctStart=Start Function (Call once and only once)  FctStart_Name=cpInitCommunications  FctStart_Declaration=inline extern void cpInitCommunications();  FctStart_Call=cpInitCommunications();  FctInit=None  FctInit_Name=Init_Reset  FctInit_Declaration=inline extern void Init_Reset();  FctInit_Call=Init_Reset();  PinDigitalInput=[]  PinDigitalOutput=[]  AnalogueInput=[]
  Load1 : Subsystem
  Master : dsPICdrivers/Master  Tag=dsPIC_MASTER  Priority=1  TimeStepType=Timer1  picType=33fJ256GP710  fcy=40000000  Quartz_33f=8e6  PLLActive_33f=on  fcyDesired_33f=40000000  tmr1="[8  49999  0]"  tmr1Info="Time Step : 0.01  ;   Error : 0%  PR1=49999"  tmr2345="[8  0  0  0  0  0  0  0]"  tmr2345cfg=[-1 -1 -1 -1 -1 -1 -1 -1]  IOautoConf=on  typePort="[ 10  10  10  10  10  10  10  10   0   0   0   0   0   0   0   0   8   0   0   0   0   0   0   0   0   8   0   8   0   0   0   0   0   0   9   0   0   0   0   0   0   0   0   0   0   0   0   0   0   7   0   0   0  10   9   9   0   6   6   6   0   9   0   6   0   0   0   0   0   0   0   0   0   0   0   0   0   0   0   0   0   0   0   0   0   0   0   0   0   0   0   0   0   0   0   0   0   0   0   9   0   0   0   0   0  10   0   0   0   0   0   0 ]"  TRIS="[ 65280  65535  65535  65501  65535  65535  65023 ]"  ADPCFG=12713984  MasterBusyPort=None  MasterOverloadPort=None  FOSC=Quartz (XT - HS)  ClockSwitchMonitor=Both disabled  TempProtection_33f=TEMP_ON  FPBOR=<empty>  PWRT=disable  MCLR=<empty>  ICD=ICS_PGD1  JTAGEN=JTAGEN_OFF  PowerSave=off  OverrideFcy=off  NewFcy=1e6  PR2345="[65535  65535  65535  65535  65535  65535  65535  65535]"
  Sensor Inputs : Subsystem
  Switch : Switch  Criteria=u2 ~= 0  OutDataType=fixdt(1, 16)  OutScaling=2^0
  Switch1 : Switch  Criteria=u2 ~= 0  OutDataType=fixdt(1, 16)  OutScaling=2^0
  Transmit actuator data : Subsystem  TreatAsAtomicUnit=on
  Transmit state data via UART1 : Subsystem
  wires:
  Sensor Inputs/1(HIL) -> [HIL]
  Sensor Inputs/2(sensors_GPS) -> [sensors_GPS]
  Sensor Inputs/3(sensors_t) -> [sensors_t]
  Sensor Inputs/4(sensors_r) -> [sensors_r]
  Sensor Inputs/5(sensors_b) -> [sensors_b]
  Controller/1(command_b) -> [command_b]
  Controller/2(command_r) -> [command_r]
  Controller/3(command_t) -> [command_t]
  [sensors_GPS] -> Controller/1(sensors_GPS)
  [sensors_t] -> Controller/2(sensors_t)
  [sensors_r] -> Controller/3(sensors_r)
  [sensors_b] -> Controller/4(sensors_b)
  [reset] -> Controller/5(reset)
  Sensor Inputs/6(timestamp) -> [timestamp]
  Sensor Inputs/7(reset) -> [reset]
  [command_r] -> Actuator Outputs/1(command_r)
  [command_t] -> Actuator Outputs/2(command_t)
  [HIL] -> Transmit actuator data/5(HIL enable)
  [command_r] -> Transmit actuator data/1(rudder)
  [command_t] -> Transmit actuator data/2(throttle)
  [command_b] -> Transmit actuator data/3(ballast)
  [timestamp] -> Transmit actuator data/4(seconds)
  Initialize UARTs [commProtocol.c]/1 -> Initialize GPS [gps.c]/1
  Initialize Data EE  emulation [DEE.c]/1 -> Initialize RC calibration ranges from NVRAM [misc.c]/1
  [HIL] -> Controller/6(HIL)
  [sensors_r] -> Actuator Outputs/3(Rudder Sensor Inputs)
  Controller/4(waypoints) -> [waypoints]
  [reset_startup] -> Bitwise-combine/1(bit0)
  [reset_GPS_discon] -> Bitwise-combine/4(bit3)
  [reset_HIL_discon] -> Bitwise-combine/3(bit2)
  [reset_HIL_toggle] -> Bitwise-combine/2(bit1)
  [reset_track] -> Bitwise-combine/5(bit4)
  [reset_calibrated] -> Bitwise-combine/6(bit5)
  [reset_calibration_mode] -> Bitwise-combine/7(bit6)
  [reset_estop] -> Bitwise-combine/8(bit7)
  Bitwise-combine/1(Out1) -> Transmit state data via UART1/7(Reset)
  [SensedGlobalPosition] -> Transmit state data via UART1/1(gPos)
  [SensedHeading] -> Transmit state data via UART1/2(head)
  [SensedLocalPosition] -> Transmit state data via UART1/3(lPos)
  [SensedVelocity] -> Transmit state data via UART1/4(vel)
  [sensors_GPS] -> Transmit state data via UART1/6(GPS)
  [sensors_r] -> Transmit state data via UART1/5(rudder)
  [rudder_angle] -> Transmit state data via UART1/9(RudderAngle)
  [v_rpm] -> Transmit state data via UART1/10(v_rpm)
  Bitwise-combine1/1(Out1) -> Transmit state data via UART1/11(status)
  Load1/1(load) -> Transmit state data via UART1/8(Load)
  [autoMode] -> Bitwise-combine1/1(bit0)
  [HILSensorsMode] -> Bitwise-combine1/2(bit1)
  [RC_Disconnected] -> Bitwise-combine1/3(bit2)
  ECAN1 Error Status/1(tx_err) -> Data Type Conversion1/1
  ECAN1 Error Status/2(rx_err) -> Data Type Conversion/1
  Constant4/1 -> Bitwise-combine1/7(bit6)
  Constant5/1 -> Bitwise-combine1/8(bit7)
  [autoMode] -> Switch/2
  [autoRudderAngleCommand] -> Switch/1
  [manualRudderAngleCommand] -> Switch/3
  Switch/1 -> Transmit state data via UART1/12(rudderAngleCommand)
  [autoMode] -> Switch1/2
  [autoThrottleCommand] -> Switch1/1
  [manualThrottleCommand] -> Switch1/3
  Switch1/1 -> Transmit state data via UART1/13(throttleCommand)
  [rudder_angle] -> Transmit actuator data/6(rudderAngle)
  [HILSensorsMode] -> Transmit actuator data/7(sensorOverride)
  Data Type Conversion/1 -> Bitwise-combine1/5(bit4)
  Data Type Conversion1/1 -> Bitwise-combine1/4(bit3)
  Constant1/1 -> Bitwise-combine1/6(bit5)
  [BatteryVoltage] -> Transmit state data via UART1/14(batteryVoltage)
  [BatteryAmperage] -> Transmit state data via UART1/15(batteryAmperage)
  [lowCalibrationLimit] -> Transmit state data via UART1/16(lowRudderCalLimit)
  [highCalibrationLimit] -> Transmit state data via UART1/17(highRudderCalLimit)

== system code_gen_HeadingHold/Actuator Outputs ==
  note: Propulsion is controlled here via a CAN interface to the motor driver board.
      | ECAN1 is used and several possible commands are transmitted: enable, disable,
      | or change speed, with speed being between -1023 and 1023 taken as a fraction
      | of total speed (1023).
  note: Rudder commands are output via a pulse-train signaling step (through the OC2 pins),
      | a direction bit set via RD5, and an enable bit set via RG9. Dir = 1 indicates port, while
      | dir = 0 indicates starboard
  command_r : Inport
  command_t : Inport  Port=2  OutDataType=fixdt(1, 16)  OutScaling=2^0
  Rudder Sensor Inputs : Inport  Port=3  OutDataType=sfix(16)  OutScaling=2^0
  Bus Selector : BusSelector  OutputSignals=enable,direction,up,period
  Bus Selector1 : BusSelector  OutputSignals=identifier,data,size,trigger
  Bus Selector2 : BusSelector  OutputSignals=limit port,limit starboard
  Constant4 : Constant  Value=0  OutDataTypeMode=uint16  OutDataType=sfix(16)  OutScaling=2^0  OutDataTypeStr=uint16
  Digital Output Write : dsPICdrivers/Digital I//O/Digital Output Write  Tag=dsPIC_Digital_Output  Priority=5  PORT=D  Pin=[5]  Simultaneous=off  OrderingInOutPopup=None
  Digital Output Write1 : dsPICdrivers/Digital I//O/Digital Output Write  Tag=dsPIC_Digital_Output  Priority=5  PORT=G  Pin=[9]  Simultaneous=off  OrderingInOutPopup=None
  Rudder Motor : dsPICdrivers/Peripheral I//O/Output Compare  Tag=dsPIC_PWM_out  Priority=5  IntPriority=3  CHANNEL=[2]  Channel_UP_Down_Periode=[5]  MaxChannel=[0.01]  MaxName=' OC2max '  Precision=[15.6096]  Timer=[2]  Status=OK  SafeMarge=[0]  PortLetter=[68]  PortNumber=[1]  MaxValues=[49999]
  Switch1 : Switch  Criteria=u2 ~= 0  Threshold=1  OutDataTypeStr=Inherit: Inherit via back propagation
  Switch2 : Switch  Criteria=u2 ~= 0  Threshold=1  OutDataTypeStr=Inherit: Inherit via back propagation
  Switch3 : Switch  Criteria=u2 ~= 0  Threshold=1  OutDataTypeStr=Inherit: Inherit via back propagation
  To Drive Motor : Subsystem  mask(Send ECAN Message){buffer=0, identifier=hex2dec('401'), identifier_from_input=on, ide=off, remote=off, data=[hex2dec('11') hex2dec('12') hex2dec('13') hex2dec('14')], data_length=4, data_from_input=on, c_func_sample_time=.01, trigger_on_input=on}
      mask prompts: identifier_from_input "Identifier from input"; data_length "Data length"; data_from_input "Data from input"; c_func_sample_time "Sample time"; trigger_on_input "Trigger on input"
      mask help: This block allows for the transmission of a message over the ECAN module.
      mask CallbackString:
      | ||mEnables = get_param(gcb,'MaskEnables');
      | enabled = get_param(gcb, 'identifier_from_input');
      | if strcmp(enabled,'on');
      |     replace_block([gcb '/identifier'],'Constant','Inport','noprompt');
      |     mEnables{2} = 'off';
      |     set_param([gcb '/identifier'],'Port','1');
      | else
      |     replace_block([gcb '/identifier'],'Inport','Constant','noprompt');
      |     mEnables{2} = 'on';
      |     set_param([gcb '/identifier'],'Value','identifier');
      | end
      | set_param(gcb, 'MaskEnables', mEnables);
      | |||data = eval(get_param(gcb, 'data'));
      | y = size(data,1);
      | x = size(data,2);
      | if y > 1 && x > 1
      |     error('Data must be a 1-dimensional vector')
      | else
      |     if or(x > 8, y > 8)
      |         error('Data cannot be larger than 8-bytes');
      |     end
      | end
      | 
      | set_param(gcb, 'data_length', num2str(length(data)));|data_length = eval(get_param(gcb, 'data_length'));
      | if or(data_length < 0, data_length > 9)
      |     error('Data cannot be more than 8 bytes or less than 0.')
      | end|mEnables = get_param(gcb,'MaskEnables');
      | enabled = get_param(gcb, 'data_from_input');
      | if strcmp(enabled,'on');
      |     replace_block([gcb '/data'],'Constant','Inport','noprompt');
      |     replace_block([gcb '/data_length'],'Constant','Inport','noprompt');
      |     mEnables{6} = 'off';
      |     mEnables{7} = 'off';
      |     port = 1;
      |     if ~isempty(find_system(gcb,'LookUnderMasks','all','Name','identifier'))
      |         port = 2;
      |     end
      |     set_param([gcb '/data'],'Port',num2str(port));
      |     set_param([gcb '/data_length'],'Port',num2str(port+1));
      | else
      |     replace_block([gcb '/data'],'Inport','Constant','noprompt');
      |     replace_block([gcb '/data_length'],'Inport','Constant','noprompt');
      |     mEnables{6} = 'on';
      |     mEnables{7} = 'on';
      |     set_param([gcb '/data'],'Value','data');
      |     set_param([gcb '/data'],'OutDataTypeMode','uint8');
      |     set_param([gcb '/data_length'],'Value','data_length');
      |     set_param([gcb '/data_length'],'OutDataTypeMode','uint8');
      | end
      | set_param(gcb, 'MaskEnables', mEnables);
      | ||mEnables = get_param(gcb,'MaskEnables');
      | enabled = get_param(gcb, 'trigger_on_input');
      | c_func_blk = find_system(gcb,'LookUnderMasks','all','FunctionName','dsPIC_C_function_Call');
      | if strcmp(enabled,'on');
      |     mEnables{9} = 'off';
      |     %set_param(c_func_blk,'SampleTime','-1');
      |     replace_block([gcb '/trigger'],'Constant','Inport','noprompt');
      | else
      |     mEnables{9} = 'on';
      |     %set_param(c_func_blk,'SampleTime','c_func_sample_time');
      |     replace_block([gcb '/trigger'],'Inport','Constant','noprompt');
      |     %set_param([gcb '/trigger'],'Value','1');
      | end
      | set_param(gcb, 'MaskEnables', mEnables);
      mask Display: disp('ECAN1 TX');
  wires:
  Bus Selector/2 -> Switch2/2, Digital Output Write/1  "<direction>"
  Bus Selector/1 -> Digital Output Write1/1  "<enable>"
  command_r/1 -> Bus Selector/1
  command_t/1 -> Bus Selector1/1
  Switch2/1 -> Switch1/2, Switch3/2
  Rudder Sensor Inputs/1 -> Bus Selector2/1
  Switch1/1 -> Rudder Motor/1
  Switch3/1 -> Rudder Motor/2
  Constant4/1 -> Switch1/1, Switch3/1
  Bus Selector/4 -> Switch3/3  "<period>"
  Bus Selector/3 -> Switch1/3  "<up>"
  Bus Selector2/1 -> Switch2/1  "<limit port>"
  Bus Selector2/2 -> Switch2/3  "<limit starboard>"
  Bus Selector1/1 -> To Drive Motor/1(identifier)  "<identifier>"
  Bus Selector1/2 -> To Drive Motor/2(data)  "<data>"
  Bus Selector1/3 -> To Drive Motor/3(data_length)  "<size>"
  Bus Selector1/4 -> To Drive Motor/4(trigger)  "<trigger>"

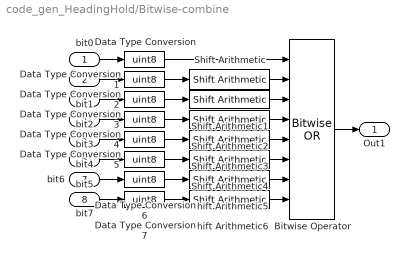
== system code_gen_HeadingHold/Bitwise-combine ==
  bit0 : Inport
  bit1 : Inport  Port=2
  bit2 : Inport  Port=3
  bit3 : Inport  Port=4
  bit4 : Inport  Port=5
  bit5 : Inport  Port=6
  bit6 : Inport  Port=7
  bit7 : Inport  Port=8
  Bitwise Operator : simulink/Logic and Bit Operations/Bitwise Operator  logicop=OR  UseBitMask=off  NumInputPorts=8  BitMask=bin2dec('11011001')  BitMaskRealWorld=Stored Integer
  Data Type Conversion{,1..7} (8 alike) : DataTypeConversion  OutDataTypeMode=uint8  OutDataType=fixdt(1, 16)  OutScaling=2^0  OutDataTypeStr=uint8
  Shift Arithmetic : simulink/Logic and Bit Operations/Shift Arithmetic  SystemSampleTime=-1  nBitShiftRight=-1  nBinPtShiftRight=0
  Shift Arithmetic1 : simulink/Logic and Bit Operations/Shift Arithmetic  SystemSampleTime=-1  nBitShiftRight=-2  nBinPtShiftRight=0
  Shift Arithmetic2 : simulink/Logic and Bit Operations/Shift Arithmetic  SystemSampleTime=-1  nBitShiftRight=-3  nBinPtShiftRight=0
  Shift Arithmetic3 : simulink/Logic and Bit Operations/Shift Arithmetic  SystemSampleTime=-1  nBitShiftRight=-4  nBinPtShiftRight=0
  Shift Arithmetic4 : simulink/Logic and Bit Operations/Shift Arithmetic  SystemSampleTime=-1  nBitShiftRight=-5  nBinPtShiftRight=0
  Shift Arithmetic5 : simulink/Logic and Bit Operations/Shift Arithmetic  SystemSampleTime=-1  nBitShiftRight=-6  nBinPtShiftRight=0
  Shift Arithmetic6 : simulink/Logic and Bit Operations/Shift Arithmetic  SystemSampleTime=-1  nBitShiftRight=-7  nBinPtShiftRight=0
  Out1 : Outport
  wires:
  Shift Arithmetic/1 -> Bitwise Operator/2
  Shift Arithmetic1/1 -> Bitwise Operator/3
  Shift Arithmetic2/1 -> Bitwise Operator/4
  Data Type Conversion/1 -> Bitwise Operator/1
  Data Type Conversion1/1 -> Shift Arithmetic/1
  Data Type Conversion2/1 -> Shift Arithmetic1/1
  Data Type Conversion3/1 -> Shift Arithmetic2/1
  Data Type Conversion4/1 -> Shift Arithmetic3/1
  Shift Arithmetic3/1 -> Bitwise Operator/5
  Data Type Conversion5/1 -> Shift Arithmetic4/1
  Data Type Conversion6/1 -> Shift Arithmetic5/1
  Shift Arithmetic4/1 -> Bitwise Operator/6
  Shift Arithmetic5/1 -> Bitwise Operator/7
  Data Type Conversion7/1 -> Shift Arithmetic6/1
  Shift Arithmetic6/1 -> Bitwise Operator/8
  bit0/1 -> Data Type Conversion/1
  bit1/1 -> Data Type Conversion1/1
  bit2/1 -> Data Type Conversion2/1
  bit3/1 -> Data Type Conversion3/1
  Bitwise Operator/1 -> Out1/1
  bit4/1 -> Data Type Conversion4/1
  bit5/1 -> Data Type Conversion5/1
  bit6/1 -> Data Type Conversion6/1
  bit7/1 -> Data Type Conversion7/1
